simulink model "pmsm_svm_control_FCN_2"  (R2019b)
settings: Solver=VariableStepAuto  StartTime=0.0  StopTime=2  MaxStep=1e-6  MinStep=1e-8  RelTol=1e-5  EnableMultiTasking=on
values from neighbouring files (symbols this model uses):
  B = 0.002    [autotune_parameters.m]    (also in siemens_400w_param.m = 2e-05)
  J = 5.8e-4    (= 0.00058)    [autotune_parameters.m]    (also in siemens_400w_param.m = 8.97e-05)
  Ld = 30e-3    (= 0.03)    [autotune_parameters.m]    (also in siemens_400w_param.m = 0.006)
  Lq = 30e-3    (= 0.03)    [autotune_parameters.m]    (also in siemens_400w_param.m = 0.006)
  pp = 4    [siemens_400w_param.m]
  Rs = 7.1    [autotune_parameters.m]    (also in siemens_400w_param.m = 4.2)
  Tf = 0    [siemens_400w_param.m]
libraries: fl_lib x8, powerlib x5, simulink x4, nesl_utility x4, sdl_lib x1, powerlib_meascontrol x1
settings Model: Creator=User  LastModifiedBy=User
settings SolverCC: MaxConsecutiveMinStep=3  ZeroCrossControl=DisableAll  ZeroCrossAlgorithm=Adaptive
settings DataIOCC: LimitDataPoints=on  SaveFormat=Array  ReturnWorkspaceOutputs=off
settings OptimizationCC: LifeSpan=inf
settings DebuggingCC: UnderspecifiedInitializationDetection=Classic  MergeDetectMultiDrivingBlocksExec=none  SolverPrmCheckMsg=warning  SFUnexpectedBacktrackingDiag=warning  SFNoUnconditionalDefaultTransitionDiag=warning  SFExecutionAtInitializationDiag=none  ArithmeticOperatorsInVariantConditions=warning
settings HardwareCC: ProdBitPerPointer=32  ProdBitPerSizeT=32  ProdBitPerPtrDiffT=32  ProdLargestAtomicFloat=None  ProdIntDivRoundTo=Undefined  ProdEndianess=Unspecified  ProdWordSize=32  ProdHWDeviceType=32-bit Generic
settings ModelReferenceCC: PropagateSignalLabelsOutOfModel=off
settings SFSimCC: SimUseLocalCustomCode=off  CustomCodeUndefinedFunction=UseInterfaceOnly
settings RTWCC: RTWUseLocalCustomCode=off
settings CodeAppCC: StateflowObjectComments=on
settings GRTTargetCC: TargetLangStandard=C89/C90 (ANSI)  GeneratePreprocessorConditionals=Disable all
settings ConfigComp: CovMetricSettings=dw  CovHtmlReporting=on  CovSaveCumulativeToWorkspaceVar=on  CovSaveSingleToWorkspaceVar=on  CovExternalEMLEnable=off
settings SimscapeCC: SimscapeNormalizeSystem=off

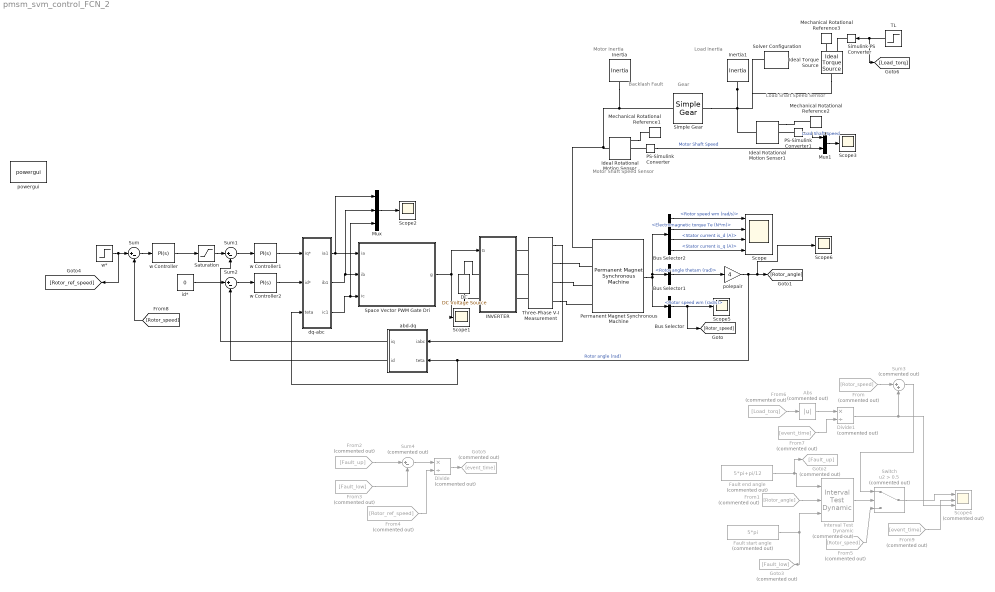
== system pmsm_svm_control_FCN_2 ==
  note: Motor Inertia
  note: Load Inertia
  note: Motor Shaft
      | Speed Sensor
  note: Load Shaft
      | Speed Sensor
  note: Gear
  note: Backlash
      | Fault
  Abs : Abs  Commented=on
  Bus Selector : BusSelector  OutputSignals=Rotor speed wm (rad/s)
  Bus Selector1 : BusSelector  OutputSignals=Rotor angle thetam (rad)
  Bus Selector2 : BusSelector  OutputSignals=Rotor speed wm (rad/s),Electromagnetic torque Te (N*m),Stator current is_d (A),Stator current is_q (A)
  DC : powerlib/Electrical Sources/DC Voltage Source  Amplitude=160  Measurements=None
      settings: SourceProductName=Simscape Electrical
  Divide : Product  Commented=on  Inputs=*/
  Divide1 : Product  Commented=on  Inputs=*/
  Fault end angle : Constant  Commented=on  Value=5*pi+pi/12
  Fault start angle : Constant  Commented=on  Value=5*pi
  From : From  Commented=on  GotoTag=Rotor_speed
  From1 : From  Commented=on  GotoTag=Rotor_angle
  From2 : From  Commented=on  GotoTag=Fault_up
  From3 : From  Commented=on  GotoTag=Fault_low
  From4 : From  Commented=on  GotoTag=Rotor_ref_speed
  From5 : From  Commented=on  GotoTag=Rotor_speed
  From6 : From  Commented=on  GotoTag=Load_torq
  From7 : From  Commented=on  GotoTag=event_time
  From9 : From  Commented=on  GotoTag=event_time
  Goto2 : Goto  Commented=on  GotoTag=Fault_up
  Goto3 : Goto  Commented=on  GotoTag=Fault_low
  Goto5 : Goto  Commented=on  GotoTag=event_time
  INVERTER : Subsystem
  Ideal Rotational Motion Sensor : fl_lib/Mechanical/Mechanical Sensors/Ideal Rotational Motion Sensor  offset=0 rad
  Ideal Rotational Motion Sensor1 : fl_lib/Mechanical/Mechanical Sensors/Ideal Rotational Motion Sensor  offset=0 rad
  Ideal Torque Source : fl_lib/Mechanical/Mechanical Sources/Ideal Torque Source
  Inertia : fl_lib/Mechanical/Rotational Elements/Inertia  inertia=8.97e-5 kg*m^2  w_specify=off  w_priority=High  w=0 rad/s  w_nominal_specify=off  w_nominal_unit=rad/s  w_nominal_value=1  t_specify=off  t_priority=None  t=0 N*m  t_nominal_specify=off  t_nominal_unit=N*m  t_nominal_value=1
  Inertia1 : fl_lib/Mechanical/Rotational Elements/Inertia  inertia=0.001 kg*m^2  w_specify=off  w_priority=High  w=0 rad/s  w_nominal_specify=off  w_nominal_unit=rad/s  w_nominal_value=1  t_specify=off  t_priority=None  t=0 N*m  t_nominal_specify=off  t_nominal_unit=N*m  t_nominal_value=1
  Interval Test Dynamic : simulink/Logic and Bit Operations/Interval Test Dynamic  Commented=on  IntervalClosedRight=on  IntervalClosedLeft=on  OutDataTypeStr=boolean
      settings: SourceProductName=Simulink  SourceProductBaseCode=SL
  Mechanical Rotational Reference1 : fl_lib/Mechanical/Rotational Elements/Mechanical Rotational Reference
  Mechanical Rotational Reference2 : fl_lib/Mechanical/Rotational Elements/Mechanical Rotational Reference
  Mechanical Rotational Reference3 : fl_lib/Mechanical/Rotational Elements/Mechanical Rotational Reference
  Mux : Mux  Inputs=3
  Mux1 : Mux  Inputs=2
  PS-Simulink Converter : nesl_utility/PS-Simulink Converter  PhysicalDomain=network_engine_domain  SubClassName=ps_output  LeftPortType=input  RightPortType=output  PseudoPeriodic=off  Frequencies=[]  Unit=inherit  AffineConversion=off
  PS-Simulink Converter1 : nesl_utility/PS-Simulink Converter  PhysicalDomain=network_engine_domain  SubClassName=ps_output  LeftPortType=input  RightPortType=output  PseudoPeriodic=off  Frequencies=[]  Unit=inherit  AffineConversion=off
  Permanent Magnet Synchronous Machine : powerlib/Machines/Permanent Magnet Synchronous Machine  NbPhases=3  FluxDistribution=Sinusoidal  RotorType=Round  MechanicalLoad=Mechanical rotational port  PresetModel=No  ShowDetailedParameters=on  MeasurementBus=off  Resistance=Rs  Inductance=8.5e-3  dqInductances=[Ld,Lq]  La=Ld  MachineConstant=Flux linkage established by magnets (V.s)  Flux=phi_magnet  VoltageCst=55.6474  TorqueCst=0.4602  Flat=120  Mechanical=[J B pp Tf]  PolePairs=4  InitialConditions=[0,0, 0,0]  InitialConditions5ph=[0 0 0 0 0 0]  RefAngle=Aligned with phase A axis (original Park)  IterativeDiscreteModel=Trapezoidal non iterative  TsBlock=-1  TsPowergui=0
  Saturation : Saturate  UpperLimit=1.27  LowerLimit=-1.27
  Scope : Scope  NumInputPorts=4
  Scope{1..3,5..6} (5 alike) : Scope
  Scope4 : Scope  Commented=on  NumInputPorts=3
  Simple Gear : sdl_lib/Gears/Simple Gear  ratio=1  rotation_direction=1  friction_model=sdl.enum.gear_efficiencies_load.off  T_noload=0.1 N*m  T_nom=5 N*m  efficiency_nom=0.8  efficiency=0.8  mu_visc=[0, 0] N*m/(rad/s)  w_thr=0.01 rad/s  pwr_thr=0.001 W  enable_faults=simscape.enum.onoff.off  efficiency_fault=0.05  external_fault=simscape.enum.onoff.off  temporal_fault=simscape.enum.onoff.off  fault_time=5 s  fault_angles=pi / 12 rad  report_fault=1  temperature_TLU=[280, 300, 320] K  load_TLU=[1, 5, 10] N*m  efficiency_TLU=[.95, .9, .85]  efficiency_TLU2=[.85, .8, .75; .95, .9, .85; .85, .8, .7]  thermal_mass=50 J/K  T_init=300 K
      settings: SourceProductName=Simscape Driveline
  Simulink-PS Converter : nesl_utility/Simulink-PS Converter  PhysicalDomain=network_engine_domain  SubClassName=ps_input  LeftPortType=input  RightPortType=output  PseudoPeriodic=off  Frequencies=[]  NoiseDistribution=none  NoiseParameters=[]  Unit=1  AffineConversion=off  FilteringAndDerivatives=provide  SimscapeFilterOrder=1  InputFilterTimeConstant=0.001  UdotUserProvided=0
  Solver Configuration : nesl_utility/Solver Configuration  PhysicalDomain=network_engine_domain  SubClassName=solver  LeftPortType=input  RightPortType=generic  Tones=[]  Harmonics=[]  SimulateNoise=off  Profile=off  UseLocalSampling=off  EnableSwitchedLinearOptims=on  FrequencyDomain=off  UseCCode=off  RelTol=0.001  AbsTol=1e-06  MinStep=1e-09  ToWorkspace=off  RevertToSquareIcSolve=off  NumHomotopyIterations=100  PhasorMode=off  PhasorModeNumHarmonics=1  DoDC=off  ResidualTolerance=1e-09  UseLocalSolver=off  LocalSolverChoice=NE_PARTITIONING_ADVANCER  LocalSolverSampleTime=0.001  DoFixedCost=off  MaxNonlinIter=3  MaxModeIter=2  LinearAlgebra=auto  EquationFormulation=NE_TIME_EF  DelaysMemoryBudget=1024  AutomaticFiltering=on  FilteringTimeConstant=0.001  PartitionStorageMethod=AS_NEEDED  PartitionMemoryBudget=1024  PartitionMethod=FAST
  Space Vector PWM Gate Dri : Subsystem
  Sum : Sum  Inputs=|+-
  Sum1 : Sum  Inputs=|+-
  Sum2 : Sum  Inputs=|+-
  Sum3 : Sum  Commented=on  Inputs=|++
  Sum4 : Sum  Commented=on  Inputs=|+-
  Switch : Switch  Commented=on  Criteria=u2 > Threshold  Threshold=0.5
  TL : Step  Before=-1  SampleTime=0
  Three-Phase V-I Measurement : powerlib/Measurements/Three-Phase V-I Measurement  VoltageMeasurement=no  SetLabelV=off  LabelV=Vabc  Vpu=off  VpuLL=off  CurrentMeasurement=yes  SetLabelI=off  LabelI=Iabc  Ipu=off  Pbase=100e6  Vbase=500e3  OutputType=Complex  PhasorSimulation=off  PSBequivalent=0
      settings: SourceProductName=Simscape Electrical
  abd-dq : Subsystem
  dq-abc : Subsystem
  id* : Constant  Value=0
  polepair : Gain  Gain=4
  powergui : powerlib/powergui  Priority=1  SimulationMode=Continuous  SampleTime=50e-6  frequency=60  Iterations=50  frequencyindice=0  Pbase=100e6  ErrMax=1e-4  UnitsV=kV  UnitsW=MW  buscounter=0  FunctionMessages=off  echomessages=off  EnableUseOfTLC=off  CurrentSourceSwitches=off  DisableSnubberDevices=off  DisableRonSwitches=off  DisableVfSwitches=off  DisplayEquations=off  AutomaticDiscreteSolvers=off  SolverType=Tustin  Interpol=off  ExternalGateDelay=off  methode=off  Ts=0  x0status=blocks  SPID=off  SwTol=0  HookPort=off  NonlinearTolerance=1e-4  nMaxIteration=100  ContinueOnMaxIteration=off  RestoreLinks=warning  ResistiveCurrentMeasurement=off  Frange=[0:2:500]  Ylog=off  Xlog=on  ShowGrid=off  save=off  variable=ZData  structure=ScopeData2  ZoomFFT=on  StartTime=0.05  cycles=10  DisplayStyle=1  fundamental=64.29  FreqAxis=on  MaxFrequency=1000  frequencyindicesteady=1  RmsSteady=1  display=off
      settings: SourceProductName=Simscape Electrical
  w Controller : simulink/Continuous/PID Controller  Controller=PI  Form=Parallel  TimeDomain=Continuous-time  SampleTime=1  IntegratorMethod=Forward Euler  FilterMethod=Forward Euler  ControllerParametersSource=internal  P=48  I=10  D=0  UseFilter=on  N=100  TunerSelectOption=Transfer Function Based (PID Tuner App)  InitialConditionSource=internal  InitialConditionForIntegrator=0  InitialConditionForFilter=0  DifferentiatorICPrevScaledInput=0  ExternalReset=none  TrackingMode=off  Kt=1  LimitOutput=off  UpperSaturationLimit=inf  LowerSaturationLimit=-inf  LinearizeAsGain=on  AntiWindupMode=none  Kb=1  POutMin=[]  POutMax=[]  IOutMin=[]  IOutMax=[]  DOutMin=[]  DOutMax=[]  NOutMin=[]  NOutMax=[]  SumOutMin=[]  SumOutMax=[]  SaturationOutMin=[]  SaturationOutMax=[]  PParamMin=[]  PParamMax=[]  IParamMin=[]  IParamMax=[]  DParamMin=[]  DParamMax=[]  NParamMin=[]  NParamMax=[]  KbParamMin=[]  KbParamMax=[]  KtParamMin=[]  KtParamMax=[]  KbOutMin=[]  KbOutMax=[]  KtOutMin=[]  KtOutMax=[]  IntegratorOutMin=[]  IntegratorOutMax=[]  FilterOutMin=[]  FilterOutMax=[]  SumI1OutMin=[]  SumI1OutMax=[]  SumI2OutMin=[]  SumI2OutMax=[]  SumI3OutMin=[]  SumI3OutMax=[]  SumI4OutMin=[]  SumI4OutMax=[]  SumDOutMin=[]  SumDOutMax=[]  DifferentiatorOutMin=[]  DifferentiatorOutMax=[]  FilterDiffOutCoefMin=[]  FilterDiffOutCoefMax=[]  ReciprocalOutMin=[]  ReciprocalOutMax=[]  SumDenOutMin=[]  SumDenOutMax=[]  SumNumOutMin=[]  SumNumOutMax=[]  DivideOutMin=[]  DivideOutMax=[]  IntegratorContinuousStateAttributes=''  IntegratorStateMustResolveToSignalObject=off  IntegratorRTWStateStorageClass=Auto  FilterContinuousStateAttributes=''  FilterStateMustResolveToSignalObject=off  FilterRTWStateStorageClass=Auto  ParallelPVariant=InternalParameters  IdealPVariant=Disabled  IVariant=InternalParameters  DVariant=Disabled  IntegratorVariant=Continuous  SatVariant=Disabled  AWVariant=Passthrough  PCopyVariant=Disabled  TRVariant=Disabled  FdbkBlocksVariant=Forward  IdealPFdbkVariant=Disabled  SatFdbkVariant=Disabled  DerivativeFilterVariant=Disabled  NVariant=Disabled  NCopyVariant=Disabled_SignalSpec  FilterICVariant=Disabled  IntegratorICVariant=InternalICs  ExternalResetVariant=Disabled  TRSumVariant=Passthrough  SumFdbkVariant=Disabled  SumVariant=Sum_PI
  w Controller1 : simulink/Continuous/PID Controller  Controller=PI  Form=Parallel  TimeDomain=Continuous-time  SampleTime=1  IntegratorMethod=Forward Euler  FilterMethod=Forward Euler  ControllerParametersSource=internal  P=18  I=3  D=5  UseFilter=on  N=100  TunerSelectOption=Transfer Function Based (PID Tuner App)  InitialConditionSource=internal  InitialConditionForIntegrator=0  InitialConditionForFilter=0  DifferentiatorICPrevScaledInput=0  ExternalReset=none  TrackingMode=off  Kt=1  LimitOutput=off  UpperSaturationLimit=inf  LowerSaturationLimit=-inf  LinearizeAsGain=on  AntiWindupMode=none  Kb=1  POutMin=[]  POutMax=[]  IOutMin=[]  IOutMax=[]  DOutMin=[]  DOutMax=[]  NOutMin=[]  NOutMax=[]  SumOutMin=[]  SumOutMax=[]  SaturationOutMin=[]  SaturationOutMax=[]  PParamMin=[]  PParamMax=[]  IParamMin=[]  IParamMax=[]  DParamMin=[]  DParamMax=[]  NParamMin=[]  NParamMax=[]  KbParamMin=[]  KbParamMax=[]  KtParamMin=[]  KtParamMax=[]  KbOutMin=[]  KbOutMax=[]  KtOutMin=[]  KtOutMax=[]  IntegratorOutMin=[]  IntegratorOutMax=[]  FilterOutMin=[]  FilterOutMax=[]  SumI1OutMin=[]  SumI1OutMax=[]  SumI2OutMin=[]  SumI2OutMax=[]  SumI3OutMin=[]  SumI3OutMax=[]  SumI4OutMin=[]  SumI4OutMax=[]  SumDOutMin=[]  SumDOutMax=[]  DifferentiatorOutMin=[]  DifferentiatorOutMax=[]  FilterDiffOutCoefMin=[]  FilterDiffOutCoefMax=[]  ReciprocalOutMin=[]  ReciprocalOutMax=[]  SumDenOutMin=[]  SumDenOutMax=[]  SumNumOutMin=[]  SumNumOutMax=[]  DivideOutMin=[]  DivideOutMax=[]  IntegratorContinuousStateAttributes=''  IntegratorStateMustResolveToSignalObject=off  IntegratorRTWStateStorageClass=Auto  FilterContinuousStateAttributes=''  FilterStateMustResolveToSignalObject=off  FilterRTWStateStorageClass=Auto  ParallelPVariant=InternalParameters  IdealPVariant=Disabled  IVariant=InternalParameters  DVariant=Disabled  IntegratorVariant=Continuous  SatVariant=Disabled  AWVariant=Passthrough  PCopyVariant=Disabled  TRVariant=Disabled  FdbkBlocksVariant=Forward  IdealPFdbkVariant=Disabled  SatFdbkVariant=Disabled  DerivativeFilterVariant=Disabled  NVariant=Disabled  NCopyVariant=Disabled_SignalSpec  FilterICVariant=Disabled  IntegratorICVariant=InternalICs  ExternalResetVariant=Disabled  TRSumVariant=Passthrough  SumFdbkVariant=Disabled  SumVariant=Sum_PI
  w Controller2 : simulink/Continuous/PID Controller  Controller=PI  Form=Parallel  TimeDomain=Continuous-time  SampleTime=1  IntegratorMethod=Forward Euler  FilterMethod=Forward Euler  ControllerParametersSource=internal  P=12  I=5  D=5  UseFilter=on  N=100  TunerSelectOption=Transfer Function Based (PID Tuner App)  InitialConditionSource=internal  InitialConditionForIntegrator=0  InitialConditionForFilter=0  DifferentiatorICPrevScaledInput=0  ExternalReset=none  TrackingMode=off  Kt=1  LimitOutput=off  UpperSaturationLimit=inf  LowerSaturationLimit=-inf  LinearizeAsGain=on  AntiWindupMode=none  Kb=1  POutMin=[]  POutMax=[]  IOutMin=[]  IOutMax=[]  DOutMin=[]  DOutMax=[]  NOutMin=[]  NOutMax=[]  SumOutMin=[]  SumOutMax=[]  SaturationOutMin=[]  SaturationOutMax=[]  PParamMin=[]  PParamMax=[]  IParamMin=[]  IParamMax=[]  DParamMin=[]  DParamMax=[]  NParamMin=[]  NParamMax=[]  KbParamMin=[]  KbParamMax=[]  KtParamMin=[]  KtParamMax=[]  KbOutMin=[]  KbOutMax=[]  KtOutMin=[]  KtOutMax=[]  IntegratorOutMin=[]  IntegratorOutMax=[]  FilterOutMin=[]  FilterOutMax=[]  SumI1OutMin=[]  SumI1OutMax=[]  SumI2OutMin=[]  SumI2OutMax=[]  SumI3OutMin=[]  SumI3OutMax=[]  SumI4OutMin=[]  SumI4OutMax=[]  SumDOutMin=[]  SumDOutMax=[]  DifferentiatorOutMin=[]  DifferentiatorOutMax=[]  FilterDiffOutCoefMin=[]  FilterDiffOutCoefMax=[]  ReciprocalOutMin=[]  ReciprocalOutMax=[]  SumDenOutMin=[]  SumDenOutMax=[]  SumNumOutMin=[]  SumNumOutMax=[]  DivideOutMin=[]  DivideOutMax=[]  IntegratorContinuousStateAttributes=''  IntegratorStateMustResolveToSignalObject=off  IntegratorRTWStateStorageClass=Auto  FilterContinuousStateAttributes=''  FilterStateMustResolveToSignalObject=off  FilterRTWStateStorageClass=Auto  ParallelPVariant=InternalParameters  IdealPVariant=Disabled  IVariant=InternalParameters  DVariant=Disabled  IntegratorVariant=Continuous  SatVariant=Disabled  AWVariant=Passthrough  PCopyVariant=Disabled  TRVariant=Disabled  FdbkBlocksVariant=Forward  IdealPFdbkVariant=Disabled  SatFdbkVariant=Disabled  DerivativeFilterVariant=Disabled  NVariant=Disabled  NCopyVariant=Disabled_SignalSpec  FilterICVariant=Disabled  IntegratorICVariant=InternalICs  ExternalResetVariant=Disabled  TRSumVariant=Passthrough  SumFdbkVariant=Disabled  SumVariant=Sum_PI
  w* : Step  Before=100  After=-100  SampleTime=0
  wires:
  Sum/1 -> w Controller/1
  w*/1 -> [Rotor_ref_speed], Sum/1
  Permanent Magnet Synchronous Machine/1 -> Bus Selector2/1, Bus Selector1/1, Bus Selector/1
  Bus Selector1/1 -> polepair/1  "<Rotor angle thetam (rad)>"
  Bus Selector2/1 -> Scope/1  "<Rotor speed wm (rad/s)>"
  Bus Selector2/2 -> Scope/2  "<Electromagnetic torque Te (N*m)>"
  Bus Selector2/3 -> Scope/3  "<Stator current is_d (A)>"
  Bus Selector2/4 -> Scope/4  "<Stator current is_q (A)>"
  w Controller/1 -> Saturation/1
  Sum1/1 -> w Controller1/1
  w Controller1/1 -> dq-abc/1(iq*)
  id*/1 -> Sum2/1
  Sum2/1 -> w Controller2/1
  w Controller2/1 -> dq-abc/2(id*)
  Three-Phase V-I Measurement/1 -> abd-dq/1(iabc)
  abd-dq/1(iq) -> Sum1/2
  abd-dq/2(id) -> Sum2/2
  dq-abc/1(ia1) -> Mux/1, Space Vector PWM Gate Dri/1(ia)
  dq-abc/2(ib1) -> Mux/2, Space Vector PWM Gate Dri/2(ib)
  dq-abc/3(ic1) -> Mux/3, Space Vector PWM Gate Dri/3(ic)
  Space Vector PWM Gate Dri/1(g) -> Scope1/1, INVERTER/1(G)
  Mux/1 -> Scope2/1
  Saturation/1 -> Sum1/1
  PS-Simulink Converter/1 -> Mux1/2  "Motor Shaft Speed"
  PS-Simulink Converter1/1 -> Mux1/1  "Load Shaft Speed"
  Mux1/1 -> Scope3/1
  Bus Selector/1 -> [Rotor_speed], Scope5/1  "<Rotor speed wm (rad/s)>"
  polepair/1 -> Scope6/1, [Rotor_angle], dq-abc/3(teta), abd-dq/2(teta)  "Rotor angle (rad)"
  Fault end angle/1 -> Goto2/1, Interval Test Dynamic/1
  Interval Test Dynamic/1 -> Switch/2
  Sum3/1 -> Switch/1
  Switch/1 -> Scope4/1
  From/1 -> Sum3/1
  From1/1 -> Interval Test Dynamic/2
  Fault start angle/1 -> Goto3/1, Interval Test Dynamic/3
  From2/1 -> Sum4/1
  From3/1 -> Sum4/2
  Sum4/1 -> Divide/1
  From4/1 -> Divide/2
  Divide/1 -> Goto5/1
  From5/1 -> Switch/3
  From6/1 -> Abs/1
  From7/1 -> Divide1/2
  [Rotor_speed] -> Sum/2
  From9/1 -> Scope4/2
  Abs/1 -> Divide1/1
  Divide1/1 -> Scope4/3, Sum3/2
  TL/1 -> [Load_torq], Simulink-PS Converter/1
  connections:
  Three-Phase V-I Measurement/LConn1 -- INVERTER/RConn1
  Three-Phase V-I Measurement/LConn2 -- INVERTER/RConn2
  Three-Phase V-I Measurement/LConn3 -- INVERTER/RConn3
  Three-Phase V-I Measurement/RConn1 -- Permanent Magnet Synchronous Machine/LConn2
  Three-Phase V-I Measurement/RConn2 -- Permanent Magnet Synchronous Machine/LConn3
  Three-Phase V-I Measurement/RConn3 -- Permanent Magnet Synchronous Machine/LConn4
  DC/RConn1 -- INVERTER/LConn1
  DC/LConn1 -- INVERTER/LConn2
  Inertia1/LConn1 -- Ideal Rotational Motion Sensor1/LConn1 -- Ideal Torque Source/LConn1 -- Solver Configuration/RConn1 -- Simple Gear/RConn1
  PS-Simulink Converter/LConn1 -- Ideal Rotational Motion Sensor/RConn2
  PS-Simulink Converter1/LConn1 -- Ideal Rotational Motion Sensor1/RConn2
  Ideal Rotational Motion Sensor1/RConn1 -- Mechanical Rotational Reference2/LConn1
  Inertia/LConn1 -- Simple Gear/LConn1 -- Permanent Magnet Synchronous Machine/LConn1 -- Ideal Rotational Motion Sensor/LConn1
  Ideal Rotational Motion Sensor/RConn1 -- Mechanical Rotational Reference1/LConn1
  Mechanical Rotational Reference3/LConn1 -- Ideal Torque Source/RConn2
  Simulink-PS Converter/RConn1 -- Ideal Torque Source/RConn1

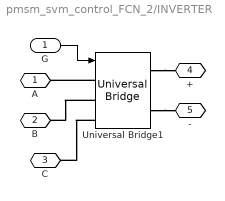
== system pmsm_svm_control_FCN_2/INVERTER ==
  G : Inport
  Universal Bridge1 : powerlib/Power Electronics/Universal Bridge  Arms=3  SnubberResistance=1e5  SnubberCapacitance=inf  Device=IGBT / Diodes  Ron=1e-3  Lon=0  ForwardVoltages="[  0  0  ]"  ForwardVoltage=0  GTOparameters=[ 10e-6 , 20e-6 ]  IGBTparameters=[ 1e-6 , 2e-6 ]  Measurements=None  Measurements_2=None  converterType=Rectifier
      settings: SourceProductName=Simscape Electrical
  A : PMIOPort  Side=Right
  B : PMIOPort  Port=2  Side=Right
  C : PMIOPort  Port=3  Side=Right
  + : PMIOPort  Port=4  Side=Left
  - : PMIOPort  Port=5  Side=Left
  wires:
  G/1 -> Universal Bridge1/1
  connections:
  Universal Bridge1/RConn2 -- -/RConn1
  Universal Bridge1/RConn1 -- +/RConn1
  Universal Bridge1/LConn3 -- C/RConn1
  Universal Bridge1/LConn2 -- B/RConn1
  Universal Bridge1/LConn1 -- A/RConn1

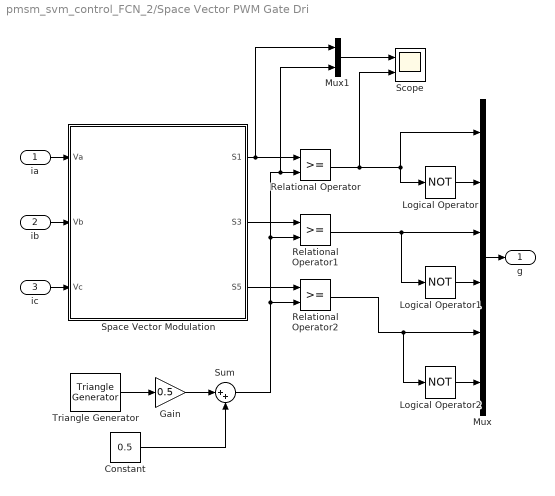
== system pmsm_svm_control_FCN_2/Space Vector PWM Gate Dri ==
  ia : Inport
  ib : Inport  Port=2
  ic : Inport  Port=3
  Constant : Constant  Value=0.5
  Gain : Gain  Gain=0.5
  Logical Operator : Logic  Operator=NOT  AllPortsSameDT=off  OutDataTypeStr=boolean
  Logical Operator1 : Logic  Operator=NOT  AllPortsSameDT=off  OutDataTypeStr=boolean
  Logical Operator2 : Logic  Operator=NOT  AllPortsSameDT=off  OutDataTypeStr=boolean
  Mux : Mux  Inputs=6
  Mux1 : Mux  Inputs=2
  Relational Operator : RelationalOperator  OutDataTypeStr=boolean  RndMeth=Nearest
  Relational Operator1 : RelationalOperator  OutDataTypeStr=boolean  RndMeth=Nearest
  Relational Operator2 : RelationalOperator  OutDataTypeStr=boolean  RndMeth=Nearest
  Scope : Scope  NumInputPorts=2
  Space Vector Modulation : Subsystem
  Sum : Sum  Inputs=|++
  Triangle Generator : powerlib_meascontrol/Pulse & Signal Generators/Triangle Generator  Freq=15000  Phase=90  Ts=0
      settings: SourceProductName=Simscape Electrical
  g : Outport
  wires:
  Logical Operator/1 -> Mux/2
  Relational Operator1/1 -> Logical Operator1/1, Mux/3
  Triangle Generator/1 -> Gain/1
  Space Vector Modulation/1(S1) -> Mux1/1, Relational Operator/1
  Space Vector Modulation/2(S3) -> Relational Operator1/1
  Space Vector Modulation/3(S5) -> Relational Operator2/1
  Mux/1 -> g/1
  Relational Operator/1 -> Scope/2, Logical Operator/1, Mux/1
  ia/1 -> Space Vector Modulation/1(Va)
  Logical Operator1/1 -> Mux/4
  Logical Operator2/1 -> Mux/6
  Relational Operator2/1 -> Logical Operator2/1, Mux/5
  ib/1 -> Space Vector Modulation/2(Vb)
  ic/1 -> Space Vector Modulation/3(Vc)
  Mux1/1 -> Scope/1
  Sum/1 -> Relational Operator2/2, Relational Operator1/2, Mux1/2, Relational Operator/2
  Constant/1 -> Sum/2
  Gain/1 -> Sum/1

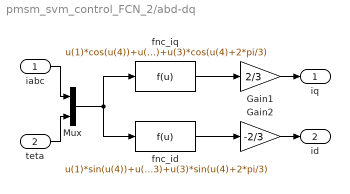
== system pmsm_svm_control_FCN_2/abd-dq ==
  iabc : Inport
  teta : Inport  Port=2
  Gain1 : Gain  Gain=2/3
  Gain2 : Gain  Gain=-2/3
  Mux : Mux  Inputs=2
  fnc_id : Fcn  Expr=u(1)*sin(u(4))+u(2)*sin(u(4)-2*pi/3)+u(3)*sin(u(4)+2*pi/3)
  fnc_iq : Fcn  Expr=u(1)*cos(u(4))+u(2)*cos(u(4)-2*pi/3)+u(3)*cos(u(4)+2*pi/3)
  iq : Outport
  id : Outport  Port=2
  wires:
  fnc_id/1 -> Gain2/1
  Gain1/1 -> iq/1
  teta/1 -> Mux/2
  iabc/1 -> Mux/1
  Mux/1 -> fnc_iq/1, fnc_id/1
  Gain2/1 -> id/1
  fnc_iq/1 -> Gain1/1

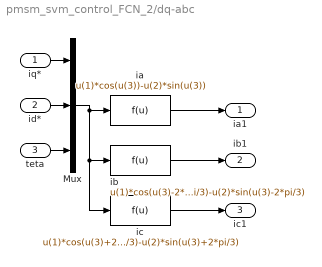
== system pmsm_svm_control_FCN_2/dq-abc ==
  iq* : Inport
  id* : Inport  Port=2
  teta : Inport  Port=3
  Mux : Mux  Inputs=3
  ia : Fcn  Expr=u(1)*cos(u(3))-u(2)*sin(u(3))
  ib : Fcn  Expr=u(1)*cos(u(3)-2*pi/3)-u(2)*sin(u(3)-2*pi/3)
  ic : Fcn  Expr=u(1)*cos(u(3)+2*pi/3)-u(2)*sin(u(3)+2*pi/3)
  ia1 : Outport
  ib1 : Outport  Port=2
  ic1 : Outport  Port=3
  wires:
  id*/1 -> Mux/2
  ia/1 -> ia1/1
  ib/1 -> ib1/1
  teta/1 -> Mux/3
  ic/1 -> ic1/1
  iq*/1 -> Mux/1
  Mux/1 -> ic/1, ib/1, ia/1

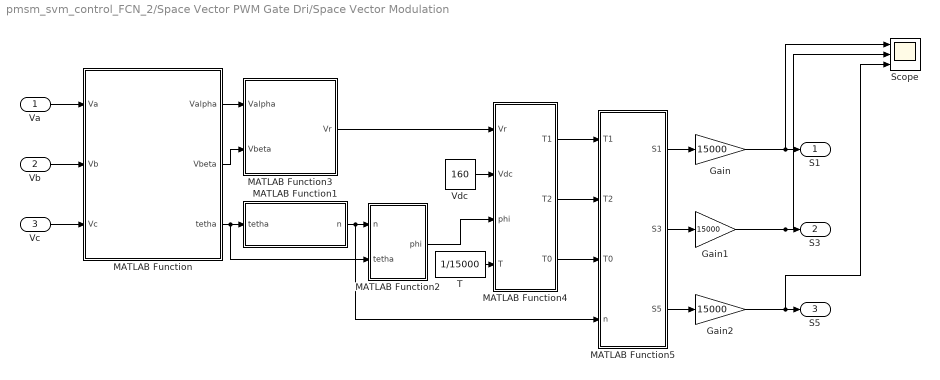
== system pmsm_svm_control_FCN_2/Space Vector PWM Gate Dri/Space Vector Modulation ==
  Va : Inport
  Vb : Inport  Port=2
  Vc : Inport  Port=3
  Gain : Gain  Gain=15000
  Gain1 : Gain  Gain=15000
  Gain2 : Gain  Gain=15000
  MATLAB Function : MATLAB Function  TreatAsAtomicUnit=on
  MATLAB Function1 : MATLAB Function  TreatAsAtomicUnit=on
  MATLAB Function2 : MATLAB Function  TreatAsAtomicUnit=on
  MATLAB Function3 : MATLAB Function  TreatAsAtomicUnit=on
  MATLAB Function4 : MATLAB Function  TreatAsAtomicUnit=on
  MATLAB Function5 : MATLAB Function  TreatAsAtomicUnit=on
  Scope : Scope  NumInputPorts=3
  T : Constant  Value=1/15000
  Vdc : Constant  Value=160
  S1 : Outport
  S3 : Outport  Port=2
  S5 : Outport  Port=3
  wires:
  MATLAB Function4/1(T1) -> MATLAB Function5/1(T1)
  MATLAB Function5/3(S5) -> Gain2/1
  MATLAB Function5/1(S1) -> Gain/1
  MATLAB Function4/2(T2) -> MATLAB Function5/2(T2)
  MATLAB Function4/3(T0) -> MATLAB Function5/3(T0)
  Va/1 -> MATLAB Function/1(Va)
  Vc/1 -> MATLAB Function/3(Vc)
  Vb/1 -> MATLAB Function/2(Vb)
  MATLAB Function/3(tetha) -> MATLAB Function2/2(tetha), MATLAB Function1/1(tetha)
  MATLAB Function1/1(n) -> MATLAB Function5/4(n), MATLAB Function2/1(n)
  MATLAB Function/1(Valpha) -> MATLAB Function3/1(Valpha)
  MATLAB Function/2(Vbeta) -> MATLAB Function3/2(Vbeta)
  MATLAB Function2/1(phi) -> MATLAB Function4/3(phi)
  MATLAB Function3/1(Vr) -> MATLAB Function4/1(Vr)
  Vdc/1 -> MATLAB Function4/2(Vdc)
  T/1 -> MATLAB Function4/4(T)
  MATLAB Function5/2(S3) -> Gain1/1
  Gain/1 -> Scope/1, S1/1
  Gain1/1 -> Scope/2, S3/1
  Gain2/1 -> Scope/3, S5/1

== matlab function pmsm_svm_control_FCN_2/Space Vector PWM Gate Dri/Space Vector Modulation/MATLAB Function1 ==
  data: tetha input; n output
function n = Sector(tetha)
n=0;
if (tetha>0)&(tetha<=pi/3)
    n=1;
end;
if (tetha>pi/3)&(tetha<=2*pi/3)
    n=2;
end;
if (tetha>2*pi/3)&(tetha<=pi)
    n=3;
end;
if (tetha<=-2*pi/3)&(tetha>-pi)
    n=4;
end;
if (tetha<=-pi/3)&(tetha>-2*pi/3)
    n=5;
end;
if (tetha<=0)&(tetha>-pi/3)
    n=6;
end;

== matlab function pmsm_svm_control_FCN_2/Space Vector PWM Gate Dri/Space Vector Modulation/MATLAB Function ==
  data: Va input; Valpha output; Vb input; Vc input; Vbeta output; tetha output
function [Valpha, Vbeta, tetha] = clark(Va, Vb, Vc)
Valpha=Va-Vb/2-Vc/2;
Vbeta=sqrt(3)/2*(Vb-Vc);
tetha=atan2(Vbeta,Valpha);

== matlab function pmsm_svm_control_FCN_2/Space Vector PWM Gate Dri/Space Vector Modulation/MATLAB Function2 ==
  data: n input; phi output; tetha input
function phi = Phi(n,tetha)
phi=0;
if (n==1)
    phi=tetha;
end;
if (n==2)
    phi=tetha-pi/3;
end;
if (n==3)
    phi=tetha-2*pi/3;
end;
if (n==4)
    phi=pi+tetha;
end;
if (n==5)
    phi=2*pi/3+tetha;
end;
if (n==6)
    phi=pi/3+tetha;
end;

== matlab function pmsm_svm_control_FCN_2/Space Vector PWM Gate Dri/Space Vector Modulation/MATLAB Function3 ==
  data: Valpha input; Vr output; Vbeta input
function Vr = Vref(Valpha,Vbeta)
Vr=sqrt(Valpha^2+Vbeta^2);

== matlab function pmsm_svm_control_FCN_2/Space Vector PWM Gate Dri/Space Vector Modulation/MATLAB Function4 ==
  data: Vr input; T1 output; Vdc input; phi input; T input; T2 output; T0 output
function [T1,T2,T0] = Timing(Vr,Vdc,phi,T)
x=Vr/Vdc;
T1=T*x*sin(pi/3-phi)/sin(pi/3);
T2=T*x*sin(phi)/sin(pi/3);
T0=T-T1-T2;

== matlab function pmsm_svm_control_FCN_2/Space Vector PWM Gate Dri/Space Vector Modulation/MATLAB Function5 ==
  data: T1 input; T2 input; T0 input; S1 output; n input; S3 output; S5 output
function [S1,S3,S5] = GATE(T1,T2,T0,n)
S1=0;
S3=0;
S5=0;
if(n==1)
    S1=T1+T2+T0/2;
    S3=T2+T0/2;
    S5=T0/2;
end;
if(n==2)
    S1=T1+T0/2;
    S3=T1+T2+T0/2;
    S5=T0/2;
end;
if(n==3)
    S1=T0/2;
    S3=T1+T2+T0/2;
    S5=T2+T0/2;
end;
if(n==4)
    S1=T0/2;
    S3=T1+T0/2;
    S5=T1+T2+T0/2;
end;
if(n==5)
    S1=T2+T0/2;
    S3=T0/2;
    S5=T1+T2+T0/2;
end;
if(n==6)
    S1=T1+T2+T0/2;
    S3=T0/2;
    S5=T1+T0/2;
end;
